simulink model "Autotrans_shift3"  (R2024a)
settings: Solver=VariableStepAuto  StartTime=0.0  StopTime=35.0  RelTol=0.001
model workspace (MATLAB code in the model file):
  | load sldemo_autotrans_data; %load initial conditions and other necessary data
undefined symbols (not defined in the file or in its folder): converter_data, downtab, emap, Hecate_brake1, Hecate_brake2, Hecate_throttle1, Hecate_throttle2, Hecate_trans, Iei, uptab, vehicledata
(part 1 of 2)
settings Model: DataTypeOverride=Off  MinMaxOverflowLogging=ForceOff  SimulationMode=accelerator  LastModifiedBy=fedformi_new
settings SolverCC: ConsecutiveZCsStepRelTol=2.8421709430404e-13
settings DataIOCC: SaveFormat=Array
settings OptimizationCC: BlockReduction=off  BooleanDataType=off  ReuseModelBlockBuffer=off
settings DebuggingCC: SaveWithParameterizedLinksMsg=none  UnderspecifiedInitializationDetection=Classic  MergeDetectMultiDrivingBlocksExec=none  SignalResolutionControl=TryResolveAllWithWarning
settings HardwareCC: TargetUnknown=on
settings ModelReferenceCC: PropagateSignalLabelsOutOfModel=off
settings RTWCC: GPUComputeCapability=3.5

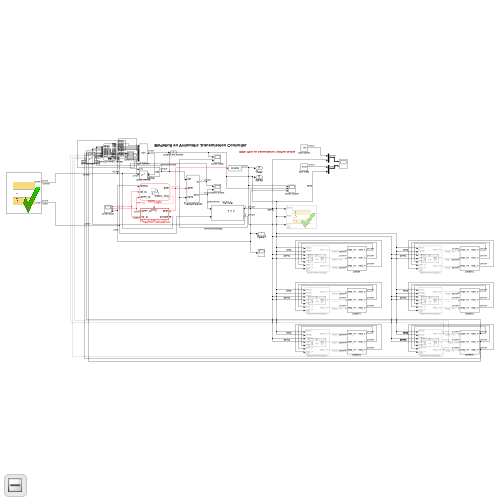
[thumbnail: Simulink's stored preview of the top-level diagram]
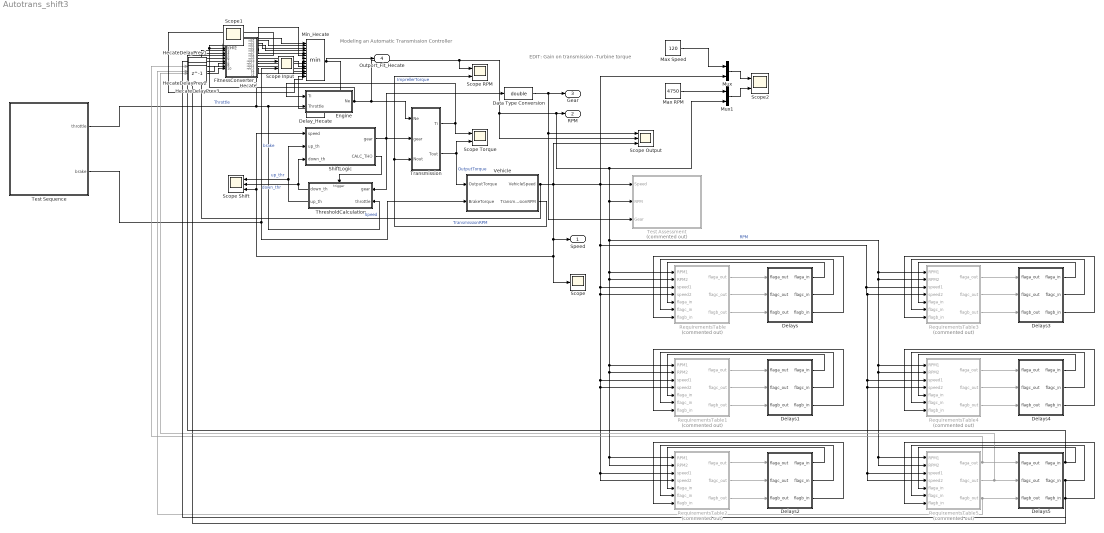
== system Autotrans_shift3 ==
  note: EDIT: Gain on transmission -Turbine torque
  note: Modeling an Automatic Transmission Controller
  Data Type Conversion : DataTypeConversion  OutDataTypeStr=double  SaturateOnIntegerOverflow=off  RndMeth=Floor
  Delay_Hecate : Delay  DelayLength=1  InitialCondition=Inf
  Delays : Subsystem
  Delays1 : Subsystem
  Delays2 : Subsystem
  Delays3 : Subsystem
  Delays4 : Subsystem
  Delays5 : Subsystem
  Engine : Subsystem
  FitnessConverter_Hecate : Stateflow chart  TreatAsAtomicUnit=on
  HecateDelayPrev1 : Delay  DelayLength=1  InitialCondition=0
  HecateDelayPrev2 : Delay  DelayLength=1  InitialCondition=0
  HecateDelayPrev3 : Delay  DelayLength=1  InitialCondition=0
  Max RPM : Constant  Value=4750
  Max Speed : Constant  Value=120
  Min_Hecate : MinMax  Inputs=14
  Mux : Mux  Inputs=2
  Mux1 : Mux  Inputs=2
  RequirementsTable : Requirements Table  Commented=on  TreatAsAtomicUnit=on
  RequirementsTable1 : Requirements Table  Commented=on  TreatAsAtomicUnit=on
  RequirementsTable2 : Requirements Table  Commented=on  TreatAsAtomicUnit=on
  RequirementsTable3 : Requirements Table  Commented=on  TreatAsAtomicUnit=on
  RequirementsTable4 : Requirements Table  Commented=on  TreatAsAtomicUnit=on
  RequirementsTable5 : Requirements Table  Commented=on  TreatAsAtomicUnit=on
  Scope : Scope
  Scope Input : Scope  NumInputPorts=2
  Scope Output : Scope  NumInputPorts=3
  Scope RPM : Scope  NumInputPorts=2
  Scope Shift : Scope  NumInputPorts=3
  Scope Torque : Scope  NumInputPorts=2
  Scope2 : Scope  NumInputPorts=2
  ShiftLogic : Stateflow chart  TreatAsAtomicUnit=on
  Test Assessment : Test Sequence  Commented=on  TreatAsAtomicUnit=on
  Test Sequence : Test Sequence  TreatAsAtomicUnit=on
  ThresholdCalculation : Subsystem  TreatAsAtomicUnit=on
  Transmission : Subsystem
  Vehicle : Subsystem  mask(vehicle model){Rfd=vehicledata(1), rload0=vehicledata(2), rload2=vehicledata(3), Rw=vehicledata(4), Iv=vehicledata(5), N20=vehicledata(6)/vehicledata(4)*vehicledata(1)}
      mask prompts: Rfd "final drive ratio"; rload0 "drag friction at wheels"; rload2 "aerodynamic drag"; Rw "wheel radius"; Iv "vehicle inertia"; N20 "initial transmission output speed"
      mask help: vehicle dynamics: torque input from trans., outputs are input speed (transmission output) and vehicle speed
      mask Display: image(imread([matlabroot,'/toolbox/simulink/simdemos/automotive/html/NSX_3Colors.jpg']))
  Speed : Outport  VectorParamsAs1DForOutWhenUnconnected=off
  RPM : Outport  Port=2  VectorParamsAs1DForOutWhenUnconnected=off
  Gear : Outport  Port=3  VectorParamsAs1DForOutWhenUnconnected=off
  Outport_Fit_Hecate : Outport  Port=4
  Scope1 : Scope
  wires:
  Transmission/1(Ti) -> Engine/1(Ti), Scope Torque/1  "ImprellerTorque"
  Vehicle/2(TransmissionRPM) -> Transmission/3(Nout), Scope RPM/2  "TransmissionRPM"
  ThresholdCalculation/1(down_th) -> Scope Shift/2, ShiftLogic/3(down_th)  "down_thr"
  ThresholdCalculation/2(up_th) -> ShiftLogic/2(up_th), Scope Shift/1  "up_thr"
  ShiftLogic/1(gear) -> Transmission/2(gear), ThresholdCalculation/1(gear), Data Type Conversion/1
  ShiftLogic/2(CALC_TH()) -> ThresholdCalculation/Trigger
  Test Sequence/1(throttle) -> Engine/2(Throttle), ThresholdCalculation/2(throttle), Scope Input/1  "Throttle"
  Transmission/2(Tout) -> Vehicle/1(OutputTorque), Scope Torque/2  "OutputTorque"
  Test Sequence/2(brake) -> Vehicle/2(BrakeTorque), Scope Input/2  "brake"
  Data Type Conversion/1 -> Scope Output/1, Test Assessment/3(Gear), Gear/1
  Mux1/1 -> Scope2/2
  Max RPM/1 -> Mux1/1
  Max Speed/1 -> Mux/1
  Mux/1 -> Scope2/1
  Delays4/1(flaga_in) -> RequirementsTable4/5(flaga_in)
  RequirementsTable1/2(flagc_out) -> Delays1/2(flagc_out)
  RequirementsTable4/2(flagc_out) -> Delays4/2(flagc_out)
  Delays4/2(flagc_in) -> RequirementsTable4/6(flagc_in)
  Delays1/2(flagc_in) -> RequirementsTable1/6(flagc_in)
  RequirementsTable4/1(flaga_out) -> Delays4/1(flaga_out)
  Vehicle/1(VehicleSpeed) -> FitnessConverter_Hecate/3(speed1), FitnessConverter_Hecate/4(speed2), Speed/1, Scope/1, Scope Shift/3, ShiftLogic/1(speed), Mux/2, Test Assessment/1(Speed), RequirementsTable3/3(speed1), RequirementsTable3/4(speed2), RequirementsTable4/3(speed1), RequirementsTable4/4(speed2), RequirementsTable5/3(speed1), RequirementsTable5/4(speed2), RequirementsTable/3(speed1), RequirementsTable/4(speed2), RequirementsTable1/3(speed1), RequirementsTable1/4(speed2), RequirementsTable2/3(speed1), RequirementsTable2/4(speed2), Scope Output/3  "Speed"
  RequirementsTable/3(flagb_out) -> Delays/3(flagb_out)
  RequirementsTable2/3(flagb_out) -> Delays2/3(flagb_out)
  RequirementsTable3/2(flagc_out) -> Delays3/2(flagc_out)
  Delays2/3(flagb_in) -> RequirementsTable2/7(flagb_in)
  RequirementsTable4/3(flagb_out) -> Delays4/3(flagb_out)
  Delays/1(flaga_in) -> RequirementsTable/5(flaga_in)
  RequirementsTable1/3(flagb_out) -> Delays1/3(flagb_out)
  Delays4/3(flagb_in) -> RequirementsTable4/7(flagb_in)
  Delays/2(flagc_in) -> RequirementsTable/6(flagc_in)
  RequirementsTable5/3(flagb_out) -> Delays5/3(flagb_out), HecateDelayPrev2/1
  Delays2/1(flaga_in) -> RequirementsTable2/5(flaga_in)
  Delays1/1(flaga_in) -> RequirementsTable1/5(flaga_in)
  RequirementsTable2/2(flagc_out) -> Delays2/2(flagc_out)
  Delays1/3(flagb_in) -> RequirementsTable1/7(flagb_in)
  RequirementsTable/2(flagc_out) -> Delays/2(flagc_out)
  RequirementsTable5/1(flaga_out) -> Delays5/1(flaga_out), HecateDelayPrev1/1
  Delays/3(flagb_in) -> RequirementsTable/7(flagb_in)
  RequirementsTable1/1(flaga_out) -> Delays1/1(flaga_out)
  RequirementsTable/1(flaga_out) -> Delays/1(flaga_out)
  Delays2/2(flagc_in) -> RequirementsTable2/6(flagc_in)
  Delays3/2(flagc_in) -> RequirementsTable3/6(flagc_in)
  RequirementsTable2/1(flaga_out) -> Delays2/1(flaga_out)
  Engine/1(Ne) -> FitnessConverter_Hecate/1(RPM1), FitnessConverter_Hecate/2(RPM2), Transmission/1(Ne), Scope RPM/1, Mux1/2, RequirementsTable3/1(RPM1), RequirementsTable3/2(RPM2), RequirementsTable4/1(RPM1), RequirementsTable4/2(RPM2), RequirementsTable5/1(RPM1), RequirementsTable5/2(RPM2), RequirementsTable/1(RPM1), RequirementsTable/2(RPM2), RequirementsTable1/1(RPM1), RequirementsTable1/2(RPM2), RequirementsTable2/1(RPM1), RequirementsTable2/2(RPM2), Test Assessment/2(RPM), RPM/1, Scope Output/2  "RPM"
  Delays5/2(flagc_in) -> RequirementsTable5/6(flagc_in), FitnessConverter_Hecate/6(flagc_in)
  Delays3/3(flagb_in) -> RequirementsTable3/7(flagb_in)
  RequirementsTable5/2(flagc_out) -> Delays5/2(flagc_out), HecateDelayPrev3/1
  Delays5/3(flagb_in) -> RequirementsTable5/7(flagb_in), FitnessConverter_Hecate/7(flagb_in)
  Delays5/1(flaga_in) -> RequirementsTable5/5(flaga_in), FitnessConverter_Hecate/5(flaga_in)
  RequirementsTable3/3(flagb_out) -> Delays3/3(flagb_out)
  RequirementsTable3/1(flaga_out) -> Delays3/1(flaga_out)
  Delays3/1(flaga_in) -> RequirementsTable3/5(flaga_in)
  HecateDelayPrev1/1 -> FitnessConverter_Hecate/8(flaga_outPrev)
  HecateDelayPrev2/1 -> FitnessConverter_Hecate/9(flagb_outPrev)
  HecateDelayPrev3/1 -> FitnessConverter_Hecate/10(flagc_outPrev)
  FitnessConverter_Hecate/1(rob1) -> Min_Hecate/1
  FitnessConverter_Hecate/2(rob2) -> Min_Hecate/2
  FitnessConverter_Hecate/3(rob3) -> Min_Hecate/3
  FitnessConverter_Hecate/4(rob4) -> Min_Hecate/4
  FitnessConverter_Hecate/5(rob5) -> Min_Hecate/5
  FitnessConverter_Hecate/6(rob6) -> Min_Hecate/6
  FitnessConverter_Hecate/7(rob7) -> Min_Hecate/7
  FitnessConverter_Hecate/8(rob8) -> Min_Hecate/8
  FitnessConverter_Hecate/9(rob9) -> Min_Hecate/9
  FitnessConverter_Hecate/10(rob10) -> Min_Hecate/10
  FitnessConverter_Hecate/11(rob11) -> Min_Hecate/11
  FitnessConverter_Hecate/12(rob12) -> Min_Hecate/12
  FitnessConverter_Hecate/13(rob13) -> Min_Hecate/13
  Min_Hecate/1 -> Delay_Hecate/1, Outport_Fit_Hecate/1
  Delay_Hecate/1 -> Min_Hecate/14

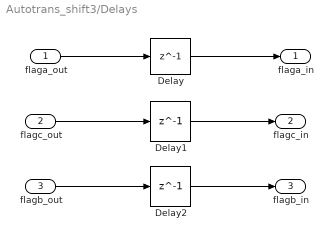
== system Autotrans_shift3/Delays ==
  flaga_out : Inport  OutDataTypeStr=boolean
  flagc_out : Inport  Port=2  OutDataTypeStr=boolean
  flagb_out : Inport  Port=3  OutDataTypeStr=boolean
  Delay : Delay  DelayLength=1  InitialCondition=false  UseCircularBuffer=on
  Delay1 : Delay  DelayLength=1  InitialCondition=false  UseCircularBuffer=on
  Delay2 : Delay  DelayLength=1  InitialCondition=false  UseCircularBuffer=on
  flaga_in : Outport  OutDataTypeStr=boolean
  flagc_in : Outport  Port=2  OutDataTypeStr=boolean
  flagb_in : Outport  Port=3  OutDataTypeStr=boolean
  wires:
  flaga_out/1 -> Delay/1
  Delay/1 -> flaga_in/1
  flagc_out/1 -> Delay1/1
  Delay1/1 -> flagc_in/1
  flagb_out/1 -> Delay2/1
  Delay2/1 -> flagb_in/1

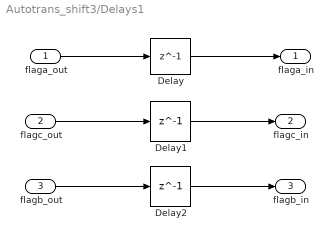
== system Autotrans_shift3/Delays1 ==
  flaga_out : Inport  OutDataTypeStr=boolean
  flagc_out : Inport  Port=2  OutDataTypeStr=boolean
  flagb_out : Inport  Port=3  OutDataTypeStr=boolean
  Delay : Delay  DelayLength=1  InitialCondition=false  UseCircularBuffer=on
  Delay1 : Delay  DelayLength=1  InitialCondition=false  UseCircularBuffer=on
  Delay2 : Delay  DelayLength=1  InitialCondition=false  UseCircularBuffer=on
  flaga_in : Outport  OutDataTypeStr=boolean
  flagc_in : Outport  Port=2  OutDataTypeStr=boolean
  flagb_in : Outport  Port=3  OutDataTypeStr=boolean
  wires:
  flaga_out/1 -> Delay/1
  Delay/1 -> flaga_in/1
  flagc_out/1 -> Delay1/1
  Delay1/1 -> flagc_in/1
  flagb_out/1 -> Delay2/1
  Delay2/1 -> flagb_in/1

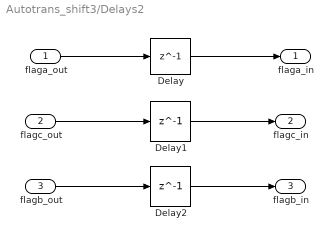
== system Autotrans_shift3/Delays2 ==
  flaga_out : Inport  OutDataTypeStr=boolean
  flagc_out : Inport  Port=2  OutDataTypeStr=boolean
  flagb_out : Inport  Port=3  OutDataTypeStr=boolean
  Delay : Delay  DelayLength=1  InitialCondition=false  UseCircularBuffer=on
  Delay1 : Delay  DelayLength=1  InitialCondition=false  UseCircularBuffer=on
  Delay2 : Delay  DelayLength=1  InitialCondition=false  UseCircularBuffer=on
  flaga_in : Outport  OutDataTypeStr=boolean
  flagc_in : Outport  Port=2  OutDataTypeStr=boolean
  flagb_in : Outport  Port=3  OutDataTypeStr=boolean
  wires:
  flaga_out/1 -> Delay/1
  Delay/1 -> flaga_in/1
  flagc_out/1 -> Delay1/1
  Delay1/1 -> flagc_in/1
  flagb_out/1 -> Delay2/1
  Delay2/1 -> flagb_in/1

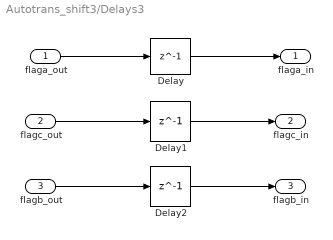
== system Autotrans_shift3/Delays3 ==
  flaga_out : Inport  OutDataTypeStr=boolean
  flagc_out : Inport  Port=2  OutDataTypeStr=boolean
  flagb_out : Inport  Port=3  OutDataTypeStr=boolean
  Delay : Delay  DelayLength=1  InitialCondition=false  UseCircularBuffer=on
  Delay1 : Delay  DelayLength=1  InitialCondition=false  UseCircularBuffer=on
  Delay2 : Delay  DelayLength=1  InitialCondition=false  UseCircularBuffer=on
  flaga_in : Outport  OutDataTypeStr=boolean
  flagc_in : Outport  Port=2  OutDataTypeStr=boolean
  flagb_in : Outport  Port=3  OutDataTypeStr=boolean
  wires:
  flaga_out/1 -> Delay/1
  Delay/1 -> flaga_in/1
  flagc_out/1 -> Delay1/1
  Delay1/1 -> flagc_in/1
  flagb_out/1 -> Delay2/1
  Delay2/1 -> flagb_in/1

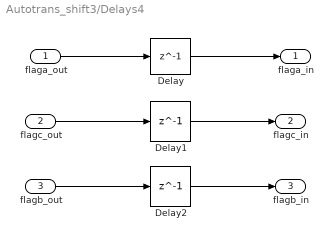
== system Autotrans_shift3/Delays4 ==
  flaga_out : Inport  OutDataTypeStr=boolean
  flagc_out : Inport  Port=2  OutDataTypeStr=boolean
  flagb_out : Inport  Port=3  OutDataTypeStr=boolean
  Delay : Delay  DelayLength=1  InitialCondition=false  UseCircularBuffer=on
  Delay1 : Delay  DelayLength=1  InitialCondition=false  UseCircularBuffer=on
  Delay2 : Delay  DelayLength=1  InitialCondition=false  UseCircularBuffer=on
  flaga_in : Outport  OutDataTypeStr=boolean
  flagc_in : Outport  Port=2  OutDataTypeStr=boolean
  flagb_in : Outport  Port=3  OutDataTypeStr=boolean
  wires:
  flaga_out/1 -> Delay/1
  Delay/1 -> flaga_in/1
  flagc_out/1 -> Delay1/1
  Delay1/1 -> flagc_in/1
  flagb_out/1 -> Delay2/1
  Delay2/1 -> flagb_in/1

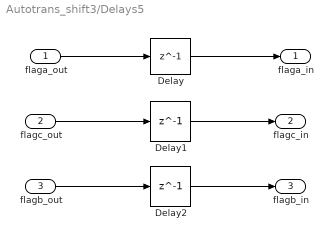
== system Autotrans_shift3/Delays5 ==
  flaga_out : Inport  OutDataTypeStr=boolean
  flagc_out : Inport  Port=2  OutDataTypeStr=boolean
  flagb_out : Inport  Port=3  OutDataTypeStr=boolean
  Delay : Delay  DelayLength=1  InitialCondition=false  UseCircularBuffer=on
  Delay1 : Delay  DelayLength=1  InitialCondition=false  UseCircularBuffer=on
  Delay2 : Delay  DelayLength=1  InitialCondition=false  UseCircularBuffer=on
  flaga_in : Outport  OutDataTypeStr=boolean
  flagc_in : Outport  Port=2  OutDataTypeStr=boolean
  flagb_in : Outport  Port=3  OutDataTypeStr=boolean
  wires:
  flaga_out/1 -> Delay/1
  Delay/1 -> flaga_in/1
  flagc_out/1 -> Delay1/1
  Delay1/1 -> flagc_in/1
  flagb_out/1 -> Delay2/1
  Delay2/1 -> flagb_in/1

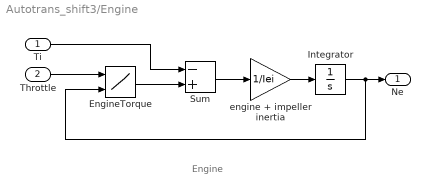
== system Autotrans_shift3/Engine ==
  note: Engine
  Ti : Inport
  Throttle : Inport  Port=2
  EngineTorque : Lookup2D  RowIndex=thvec  ColumnIndex=nevec  Table=emap  SaturateOnIntegerOverflow=off
  Integrator : Integrator  InitialCondition=1000  LimitOutput=on  UpperSaturationLimit=6000  LowerSaturationLimit=600  ZeroCross=off
  Sum : Sum  Inputs=-+  InputSameDT=on  SaturateOnIntegerOverflow=on  OutDataTypeStr=Inherit: Same as first input
  engine + impeller inertia : Gain  Gain=1/Iei  SaturateOnIntegerOverflow=on  OutDataTypeStr=Inherit: Same as input  ParamDataTypeStr=Inherit: Same as input
  Ne : Outport  InitialOutput=0  VectorParamsAs1DForOutWhenUnconnected=off
  wires:
  Ti/1 -> Sum/1
  Throttle/1 -> EngineTorque/1
  Integrator/1 -> EngineTorque/2, Ne/1
  Sum/1 -> engine + impeller inertia/1
  engine + impeller inertia/1 -> Integrator/1
  EngineTorque/1 -> Sum/2

== system Autotrans_shift3/ThresholdCalculation ==
  note: Threshold Calculation
  gear : Inport
  throttle : Inport  Port=2
  run : TriggerPort  TriggerType=function-call  VariantControl=(inherit)  ZeroCross=off
  interp_down : Lookup2D  RowIndex=downth  ColumnIndex=[1:4]  Table=downtab  OutDataTypeStr=double  SaturateOnIntegerOverflow=off  InputSameDT=off
      settings: LockScale=on
  interp_up : Lookup2D  RowIndex=upth  ColumnIndex=[1:4]  Table=uptab  OutDataTypeStr=double  SaturateOnIntegerOverflow=off  InputSameDT=off
      settings: LockScale=on
  down_th : Outport  VectorParamsAs1DForOutWhenUnconnected=off
  up_th : Outport  Port=2  VectorParamsAs1DForOutWhenUnconnected=off
  wires:
  interp_up/1 -> up_th/1
  interp_down/1 -> down_th/1
  throttle/1 -> interp_up/1, interp_down/1
  gear/1 -> interp_up/2, interp_down/2

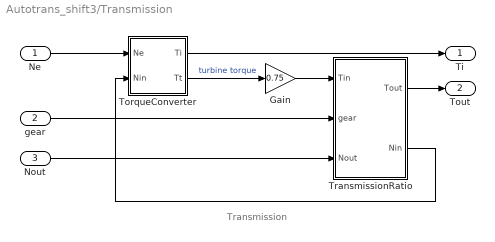
== system Autotrans_shift3/Transmission ==
  note: Transmission
  Ne : Inport
  gear : Inport  Port=2
  Nout : Inport  Port=3
  Gain : Gain  Gain=0.75
  TorqueConverter : Subsystem  mask(torque converter){speedratio=converter_data(:,1), Kfactor=converter_data(:,2), Torkratio=converter_data(:,3)}
      mask prompts: speedratio "speed ratio"; Kfactor "K factor"; Torkratio "torque ratio"
      mask help: torque converter
      mask Help: Torque converter input and output torques are computed as a function of the input and output speeds
      mask Display: plot([cos([90:10:450]*pi/180),.63*cos([90:10:450]*pi/180),.63*cos([90:10:240]*pi/180),cos([240:10:300]*pi/180),.63*cos([300]*pi/180)],[sin([90:10:450]*pi/180),.63*sin([90:10:450]*pi/180)+.1,.63*sin([90:10:240]*pi/180)+.1,sin([240:10:300]*pi/180),.63*sin([300]*pi/180)+.1])
  TransmissionRatio : Subsystem
  Ti : Outport  InitialOutput=0  VectorParamsAs1DForOutWhenUnconnected=off
  Tout : Outport  Port=2  InitialOutput=0  VectorParamsAs1DForOutWhenUnconnected=off
  wires:
  TransmissionRatio/1(Tout) -> Tout/1
  TorqueConverter/1(Ti) -> Ti/1
  Nout/1 -> TransmissionRatio/3(Nout)
  gear/1 -> TransmissionRatio/2(gear)
  Ne/1 -> TorqueConverter/1(Ne)
  TransmissionRatio/2(Nin) -> TorqueConverter/2(Nin)
  TorqueConverter/2(Tt) -> Gain/1  "turbine torque"
  Gain/1 -> TransmissionRatio/1(Tin)

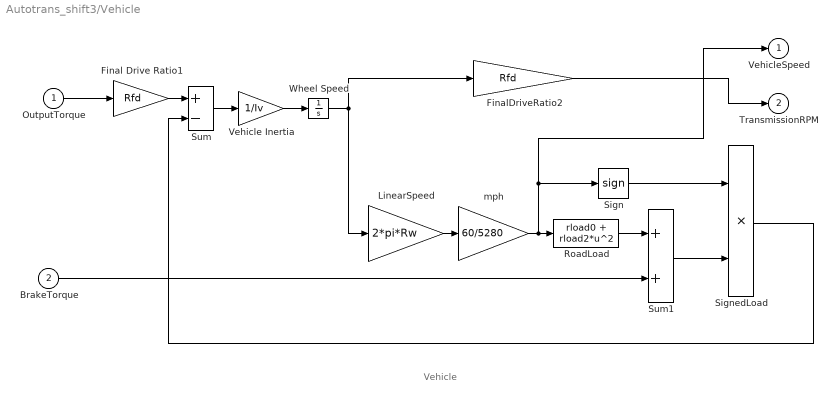
== system Autotrans_shift3/Vehicle ==
  note: Vehicle
  OutputTorque : Inport
  BrakeTorque : Inport  Port=2
  Final Drive Ratio1 : Gain  Gain=Rfd  SaturateOnIntegerOverflow=on  OutDataTypeStr=Inherit: Same as input  ParamDataTypeStr=Inherit: Same as input
  FinalDriveRatio2 : Gain  Gain=Rfd  SaturateOnIntegerOverflow=on  OutDataTypeStr=Inherit: Same as input  ParamDataTypeStr=Inherit: Same as input
  LinearSpeed : Gain  Gain=2*pi*Rw  SaturateOnIntegerOverflow=on  OutDataTypeStr=Inherit: Same as input  ParamDataTypeStr=Inherit: Same as input
  RoadLoad : Fcn  Expr=rload0 + rload2*u^2
  Sign : Signum
  SignedLoad : Product  InputSameDT=on  SaturateOnIntegerOverflow=on  OutDataTypeStr=Inherit: Same as first input
  Sum : Sum  Inputs=+-  InputSameDT=on  SaturateOnIntegerOverflow=on  OutDataTypeStr=Inherit: Same as first input
  Sum1 : Sum  InputSameDT=on  SaturateOnIntegerOverflow=on  OutDataTypeStr=Inherit: Same as first input
  Vehicle Inertia : Gain  Gain=1/Iv  SaturateOnIntegerOverflow=on  OutDataTypeStr=Inherit: Same as input  ParamDataTypeStr=Inherit: Same as input
  Wheel Speed : Integrator  InitialCondition=N20/Rfd  ZeroCross=off
  mph : Gain  Gain=60/5280  SaturateOnIntegerOverflow=on  OutDataTypeStr=Inherit: Same as input  ParamDataTypeStr=Inherit: Same as input
  VehicleSpeed : Outport  InitialOutput=0  VectorParamsAs1DForOutWhenUnconnected=off
  TransmissionRPM : Outport  Port=2  InitialOutput=0  VectorParamsAs1DForOutWhenUnconnected=off
  wires:
  FinalDriveRatio2/1 -> TransmissionRPM/1
  BrakeTorque/1 -> Sum1/2
  Sum1/1 -> SignedLoad/2
  RoadLoad/1 -> Sum1/1
  Sign/1 -> SignedLoad/1
  SignedLoad/1 -> Sum/2
  OutputTorque/1 -> Final Drive Ratio1/1
  Vehicle Inertia/1 -> Wheel Speed/1
  Sum/1 -> Vehicle Inertia/1
  mph/1 -> VehicleSpeed/1, Sign/1, RoadLoad/1
  LinearSpeed/1 -> mph/1
  Wheel Speed/1 -> LinearSpeed/1, FinalDriveRatio2/1
  Final Drive Ratio1/1 -> Sum/1

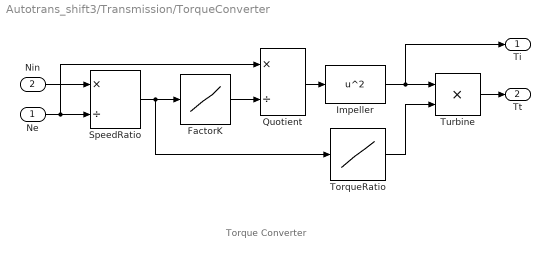
== system Autotrans_shift3/Transmission/TorqueConverter ==
  note: Torque Converter
  Ne : Inport
  Nin : Inport  Port=2
  FactorK : Lookup  InputValues=speedratio  Table=Kfactor
  Impeller : Fcn  Expr=u^2
  Quotient : Product  Inputs=*/  InputSameDT=on  SaturateOnIntegerOverflow=on  OutDataTypeStr=Inherit: Same as first input
  SpeedRatio : Product  Inputs=*/  InputSameDT=on  SaturateOnIntegerOverflow=on  OutDataTypeStr=Inherit: Same as first input
  TorqueRatio : Lookup  InputValues=speedratio  Table=Torkratio
  Turbine : Product  InputSameDT=on  SaturateOnIntegerOverflow=on  OutDataTypeStr=Inherit: Same as first input
  Ti : Outport  InitialOutput=0  VectorParamsAs1DForOutWhenUnconnected=off
  Tt : Outport  Port=2  InitialOutput=0  VectorParamsAs1DForOutWhenUnconnected=off
  wires:
  TorqueRatio/1 -> Turbine/2
  Quotient/1 -> Impeller/1
  FactorK/1 -> Quotient/2
  SpeedRatio/1 -> TorqueRatio/1, FactorK/1
  Impeller/1 -> Turbine/1, Ti/1
  Turbine/1 -> Tt/1
  Ne/1 -> SpeedRatio/2, Quotient/1
  Nin/1 -> SpeedRatio/1

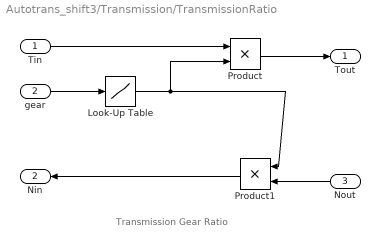
== system Autotrans_shift3/Transmission/TransmissionRatio ==
  note: Transmission Gear Ratio
  Tin : Inport
  gear : Inport  Port=2
  Nout : Inport  Port=3
  Look-Up Table : Lookup  InputValues=[1 2 3 4]  Table=[2.393 1.450 1.000 0.677]  OutDataTypeStr=double  LockScale=on
  Product : Product  InputSameDT=on  SaturateOnIntegerOverflow=on  OutDataTypeStr=Inherit: Same as first input
  Product1 : Product  InputSameDT=on  SaturateOnIntegerOverflow=on  OutDataTypeStr=Inherit: Same as first input
  Tout : Outport  InitialOutput=0  VectorParamsAs1DForOutWhenUnconnected=off
  Nin : Outport  Port=2  InitialOutput=0  VectorParamsAs1DForOutWhenUnconnected=off
  wires:
  Look-Up Table/1 -> Product1/1, Product/2
  Nout/1 -> Product1/2
  Product1/1 -> Nin/1
  Product/1 -> Tout/1
  Tin/1 -> Product/1
  gear/1 -> Look-Up Table/1

== stateflow chart Autotrans_shift3/ShiftLogic ==
  settings: updateMethod=DISCRETE  sampleTime=0.04
  state gear_state [parallel]
    settings: executionOrder=1
    state fourth
      entry:
      gear = 4;
    state third
      entry:
      gear = 3;
    state second
      entry:
      gear = 2;
    state first
      entry:
      gear = 1;
    (default) -> first
    second -> third [order 1] : UP
    first -> second : UP
    third -> fourth [order 1] : UP
    second -> first [order 2] : DOWN
    fourth -> third : DOWN
    third -> second [order 2] : DOWN
  state selection_state [parallel]
    during: CALC_TH;
    settings: executionOrder=2
    state steady_state
    state upshifting
    state downshifting
    (default) -> steady_state
    steady_state -> upshifting [order 1] : [speed > up_th]
    steady_state -> downshifting [order 2] : [speed < down_th]
    downshifting -> steady_state [order 1] : after(TWAIT,tick)
        | [speed <= down_th]
        | {gear_state.DOWN;}
    downshifting -> steady_state [order 2] : [speed > down_th]
    upshifting -> steady_state [order 1] : after(TWAIT,tick)
        | [speed >= up_th]
        | {gear_state.UP;}
    upshifting -> steady_state [order 2] : [speed < up_th]
  data: speed input double; gear output fixdt(0,8,5) [1..4]; TWAIT parameter fixdt(0,8,6); up_th input double; down_th input double
  events: DOWN local EITHER_EDGE_EVENT; UP local EITHER_EDGE_EVENT; CALC_TH output FUNCTION_CALL_EVENT

== stateflow chart Autotrans_shift3/Test Assessment ==
  state AT1
    state step_1
      state step_1_1
        verify(Speed < 120);
        settings: description=|
            | the value of the speed between [0,20]s
            | shall be lower than 120mph
      state step_1_2
      AT1.step_1 -> (junction 405)
      (default) -> (junction 405)
      (junction 405) -> (junction 406) [order 1] : [((t>=0) && (t<=20))
          | ]
      (junction 406) -> AT1.step_1.step_1_1 [order 1] : [~in(AT1.step_1.step_1_1)]
      (junction 406) -> (junction 409) [order 2]
      (junction 725) -> (junction 726)
      (junction 726) -> AT1.step_1.step_1_2 [order 1] : [~in(AT1.step_1.step_1_2)]
      (junction 726) -> (junction 729) [order 2]
      (junction 405) -> (junction 725) [order 2]
    (default) -> AT1.step_1
  state AT2
    state step_1
      state step_1_1
        verify(RPM<4750, 'Message')
      state step_1_2
      (default) -> (junction 433)
      AT2.step_1 -> (junction 433)
      (junction 433) -> (junction 434) [order 1] : [(t>=0 && t<=10)
          | ]
      (junction 434) -> AT2.step_1.step_1_1 [order 1] : [~in(AT2.step_1.step_1_1)]
      (junction 433) -> (junction 733) [order 2]
      (junction 434) -> (junction 437) [order 2]
      (junction 733) -> (junction 734)
      (junction 734) -> AT2.step_1.step_1_2 [order 1] : [~in(AT2.step_1.step_1_2)]
      (junction 734) -> (junction 737) [order 2]
    (default) -> AT2.step_1
  state AT51
    state step_1
    state AT51
      settings: description=Trigger upon changing to gear 1
    state AT51_1
      verify(Gear==1)
    (default) -> AT51.step_1
    AT51.AT51 -> AT51_1 : [
        | (hasChangedTo(Gear,1) && t>=0 && t<=30)
        | ]
    AT51_1 -> AT51.AT51 : [
        | et > 2.5
        | ]
    AT51.step_1 -> AT51.AT51 : [
        | Gear~=1
        | ]
  state AT52
    state AT52
      settings: description=Trigger upon changing to gear 2
    state AT52_1
      verify(Gear==2)
    (default) -> AT52.AT52
    AT52.AT52 -> AT52_1 : [
        | (hasChangedTo(Gear,2) && t>=0 && t<=30)
        | ]
    AT52_1 -> AT52.AT52 : [
        | et > 2.5
        | ]
  state AT53
    state AT53
      settings: description=Trigger upon changing to gear 3
    state AT53_1
      verify(Gear==3)
    (default) -> AT53.AT53
    AT53.AT53 -> AT53_1 : [
        | (hasChangedTo(Gear,3) && t>=0 && t<=30)
        | ]
    AT53_1 -> AT53.AT53 : [
        | et > 2.5
        | ]
  state AT54
    state AT54
      settings: description=Trigger upon changing to gear 4
    state AT54_1
      verify(Gear==4)
    (default) -> AT54.AT54
    AT54.AT54 -> AT54_1 : [
        | (hasChangedTo(Gear,4) && t>=0 && t<=30)
        | ]
    AT54_1 -> AT54.AT54 : [
        | et > 2.5
        | ]
  state AT6a
    state step_1
    state step_2_Inconclusive
    state step_3
    state step_4
    state step_5
      verify(true)
      settings: description=robustness calculation
    state step_6
      verify(false)
    (default) -> AT6a.step_1
    AT6a.step_1 -> (junction 589) [order 2] : [
        | ~(Speed<35)
        | ]
    (junction 589) -> (junction 587)
    AT6a.step_1 -> (junction 593) [order 3] : [
        | t>=4
        | ]
    (junction 593) -> (junction 591)
    AT6a.step_1 -> AT6a.step_2_Inconclusive [order 1] : [
        | ~(RPM<3000)
        | ]
    (junction 608) -> AT6a.step_2_Inconclusive
    (junction 610) -> (junction 608)
    AT6a.step_3 -> AT6a.step_2_Inconclusive [order 1] : [
        | ~(RPM<3000)
        | ]
    (junction 587) -> AT6a.step_3
    AT6a.step_3 -> (junction 758) [order 2] : [
        | t>=30
        | ]
    (junction 758) -> (junction 601)
    AT6a.step_4 -> (junction 610) [order 1] : [
        | ~(RPM<3000)
        | ]
    (junction 591) -> AT6a.step_4
    AT6a.step_4 -> (junction 619) [order 2] : [
        | t>=30
        | ]
    (junction 619) -> (junction 612)
    (junction 601) -> AT6a.step_5
    (junction 612) -> AT6a.step_6
  state AT6b
    state step_1
    state step_2_Inconclusive
    state step_3
    state step_4
    state step_5
      verify(true)
    state step_6
      verify(false)
    AT6b.step_4 -> (junction 658) [order 2] : [
        | t>=30
        | ]
    (default) -> AT6b.step_1
    AT6b.step_1 -> (junction 634) [order 2] : [
        | ~(Speed<50)
        | ]
    (junction 634) -> (junction 632)
    AT6b.step_1 -> (junction 641) [order 3] : [
        | t>=8
        | ]
    (junction 641) -> (junction 639)
    AT6b.step_1 -> AT6b.step_2_Inconclusive [order 1] : [
        | ~(RPM<3000)
        | ]
    (junction 644) -> AT6b.step_2_Inconclusive
    (junction 646) -> (junction 644)
    AT6b.step_3 -> AT6b.step_2_Inconclusive [order 1] : [
        | ~(RPM<3000)
        | ]
    (junction 632) -> AT6b.step_3
    AT6b.step_3 -> (junction 652) [order 2] : [
        | t>=30
        | ]
    (junction 652) -> (junction 650)
    AT6b.step_4 -> (junction 646) [order 1] : [
        | ~(RPM<3000)
        | ]
    (junction 639) -> AT6b.step_4
    (junction 650) -> AT6b.step_5
    (junction 656) -> AT6b.step_6
    (junction 658) -> (junction 656)
  state AT6c
    state step_1
    state step_2_Inconclusive
    state step_3
    state step_4
    state step_5
      verify(true)
    state step_6
      verify(false)
    AT6c.step_4 -> (junction 698) [order 2] : [
        | t>=30
        | ]
    (default) -> AT6c.step_1
    AT6c.step_1 -> (junction 674) [order 2] : [
        | ~(Speed<65)
        | ]
    (junction 674) -> (junction 672)
    AT6c.step_1 -> (junction 681) [order 3] : [
        | t>=20
        | ]
    (junction 681) -> (junction 679)
    AT6c.step_1 -> AT6c.step_2_Inconclusive [order 1] : [
        | ~(RPM<3000)
        | ]
    (junction 684) -> AT6c.step_2_Inconclusive
    (junction 686) -> (junction 684)
    AT6c.step_3 -> AT6c.step_2_Inconclusive [order 1] : [
        | ~(RPM<3000)
        | ]
    (junction 672) -> AT6c.step_3
    AT6c.step_3 -> (junction 692) [order 2] : [
        | t>=30
        | ]
    (junction 692) -> (junction 690)
    AT6c.step_4 -> (junction 686) [order 1] : [
        | ~(RPM<3000)
        | ]
    (junction 679) -> AT6c.step_4
    (junction 690) -> AT6c.step_5
    (junction 696) -> AT6c.step_6
    (junction 698) -> (junction 696)
  (default) -> AT1 [order 1] : [Active_Scenario_Index == 1]
  (default) -> AT2 [order 2] : [Active_Scenario_Index == 2]
  (default) -> AT51 [order 3] : [Active_Scenario_Index == 3]
  (default) -> AT52 [order 4] : [Active_Scenario_Index == 4]
  (default) -> AT53 [order 5] : [Active_Scenario_Index == 5]
  (default) -> AT54 [order 6] : [Active_Scenario_Index == 6]
  (default) -> AT6a [order 7] : [Active_Scenario_Index == 7]
  (default) -> AT6b [order 8] : [Active_Scenario_Index == 8]
  (default) -> AT6c [order 9] : {assert(Active_Scenario_Index == 9,'The value of Scenario Parameter ''Active_Scenario_Index'' is not valid. Use the index of the scenario to specify it.')}
  data: Speed input; RPM input; Gear input; Active_Scenario_Index parameter =1

== stateflow chart Autotrans_shift3/RequirementsTable1 ==
  (default) -> (junction 1073744871)
  (junction 1073744871) -> (junction 1073744872) : {
      | % SF_REQ_REV_07
      | }
  (junction 1073744872) -> (junction 1073744874) : {
      | % ExcEvals:
      | % PriEvals:
      | }
  (junction 1073744874) -> (junction 1073744876) : {
      | % HEADER_ASSIGNMENTS
      |
      | }
  (junction 1073744876) -> (junction 1073744878) : {
      | % START_A_4
      | }
  (junction 1073744878) -> (junction 1073744880) : {
      | }
  (junction 1073744880) -> (junction 1073744882)
  (junction 1073744882) -> (junction 1073744884) : {
      | }
  (junction 1073744884) -> (junction 1073744886) : {
      | % END_A_4
      | }
  (junction 1073744886) -> (junction 1073744888) : {
      | % START_R_7
      | }
  (junction 1073744888) -> (junction 1073744890) : {
      | }
  (junction 1073744890) -> (junction 1073744892)
  (junction 1073744892) -> (junction 1073744894) [order 1] : [(((t) >= (0) && (t) <= (20)))]
  (junction 1073744892) -> (junction 1073744900) [order 2]
  (junction 1073744894) -> (junction 1073744896) : {
      | reqtable_postcondition(((speed2)/115 < 1), 'R:1');
      |
      |
      |
      |
      | }
  (junction 1073744896) -> (junction 1073744898) : {
      | }
  (junction 1073744898) -> (junction 1073744900)
  (junction 1073744900) -> (junction 1073744902)
  (junction 1073744902) -> (junction 1073744904) : {
      | % END_R_7
      | }
  (junction 1073744904) -> (junction 1073744906) : {
      | % START_R_19
      | }
  (junction 1073744906) -> (junction 1073744908) : {
      | }
  (junction 1073744908) -> (junction 1073744910)
  (junction 1073744910) -> (junction 1073744912) [order 1] : [(((t) >= (0) && (t) <= (10)))]
  (junction 1073744910) -> (junction 1073744918) [order 2]
  (junction 1073744912) -> (junction 1073744914) : {
      | reqtable_postcondition(((RPM2)/4750 < 1), 'R:2');
      |
      |
      |
      |
      | }
  (junction 1073744914) -> (junction 1073744916) : {
      | }
  (junction 1073744916) -> (junction 1073744918)
  (junction 1073744918) -> (junction 1073744920)
  (junction 1073744920) -> (junction 1073744922) : {
      | % END_R_19
      | }
  (junction 1073744922) -> (junction 1073744924) : {
      | % START_R_34
      | }
  (junction 1073744924) -> (junction 1073744926) : {
      | }
  (junction 1073744926) -> (junction 1073744928)
  (junction 1073744928) -> (junction 1073744930) [order 1] : [((t) == 0)]
  (junction 1073744928) -> (junction 1073744936) [order 2]
  (junction 1073744930) -> (junction 1073744932) : {
      | flaga_out = true;
      | flagb_out = true;
      | flagc_out = true;
      |
      | }
  (junction 1073744932) -> (junction 1073744934) : {
      | }
  (junction 1073744934) -> (junction 1073744936)
  (junction 1073744936) -> (junction 1073744938)
  (junction 1073744938) -> (junction 1073744940) : {
      | % END_R_34
      | }
  (junction 1073744940) -> (junction 1073744942) : {
      | % START_R_22
      | }
  (junction 1073744942) -> (junction 1073744944) : {
      | }
  (junction 1073744944) -> (junction 1073744946)
  (junction 1073744946) -> (junction 1073744948) [order 1] : [(((t) <= (4))) && (speed1 >= 32)]
  (junction 1073744946) -> (junction 1073744954) [order 2]
  (junction 1073744948) -> (junction 1073744950) : {
      | flaga_out = false
      |
      |
      |
      | }
  (junction 1073744950) -> (junction 1073744952) : {
      | }
  (junction 1073744952) -> (junction 1073744954)
  (junction 1073744954) -> (junction 1073744956)
  (junction 1073744956) -> (junction 1073744958) : {
      | % END_R_22
      | }
  (junction 1073744958) -> (junction 1073744960) : {
      | % START_R_67
      | }
  (junction 1073744960) -> (junction 1073744962) : {
      | }
  (junction 1073744962) -> (junction 1073744964)
  (junction 1073744964) -> (junction 1073744966) [order 1] : [((t) > 4 || ((t) > 0 && speed1 < 32))]
  (junction 1073744964) -> (junction 1073744972) [order 2]
  (junction 1073744966) -> (junction 1073744968) : {
      | flaga_out = prev(flaga_out);
      |
      |
      |
      | }
  (junction 1073744968) -> (junction 1073744970) : {
      | }
  (junction 1073744970) -> (junction 1073744972)
  (junction 1073744972) -> (junction 1073744974)
  (junction 1073744974) -> (junction 1073744976) : {
      | % END_R_67
      | }
  (junction 1073744976) -> (junction 1073744978) : {
      | % START_R_52
      | }
  (junction 1073744978) -> (junction 1073744980) : {
      | }
  (junction 1073744980) -> (junction 1073744982)
  (junction 1073744982) -> (junction 1073744984) [order 1] : [duration((((t) <= (30))) && (RPM1 < 2900)) >= 30]
  (junction 1073744982) -> (junction 1073744990) [order 2]
  (junction 1073744984) -> (junction 1073744986) : {
      | reqtable_postcondition((((flaga_in) == (true))), 'R:6');
      |
      |
      |
      |
      | }
  (junction 1073744986) -> (junction 1073744988) : {
      | }
  (junction 1073744988) -> (junction 1073744990)
  (junction 1073744990) -> (junction 1073744992)
  (junction 1073744992) -> (junction 1073744994) : {
      | % END_R_52
      | }
  (junction 1073744994) -> (junction 1073744996) : {
      | % START_R_16
      | }
  (junction 1073744996) -> (junction 1073744998) : {
      | }
  (junction 1073744998) -> (junction 1073745000)
  (junction 1073745000) -> (junction 1073745002) [order 1] : [(((t) <= (8))) && (speed1 >= 50)]
  (junction 1073745000) -> (junction 1073745008) [order 2]
  (junction 1073745002) -> (junction 1073745004) : {
      |
      | flagb_out = false;
      |
      |
      | }
  (junction 1073745004) -> (junction 1073745006) : {
      | }
  (junction 1073745006) -> (junction 1073745008)
  (junction 1073745008) -> (junction 1073745010)
  (junction 1073745010) -> (junction 1073745012) : {
      | % END_R_16
      | }
  (junction 1073745012) -> (junction 1073745014) : {
      | % START_R_70
      | }
  (junction 1073745014) -> (junction 1073745016) : {
      | }
  (junction 1073745016) -> (junction 1073745018)
  (junction 1073745018) -> (junction 1073745020) [order 1] : [((t) > 8 || ((t) > 0 && speed1 < 50))]
  (junction 1073745018) -> (junction 1073745026) [order 2]
  (junction 1073745020) -> (junction 1073745022) : {
      |
      | flagb_out = prev(flagb_out);
      |
      |
      | }
  (junction 1073745022) -> (junction 1073745024) : {
      | }
  (junction 1073745024) -> (junction 1073745026)
  (junction 1073745026) -> (junction 1073745028)
  (junction 1073745028) -> (junction 1073745030) : {
      | % END_R_70
      | }
  (junction 1073745030) -> (junction 1073745032) : {
      | % START_R_55
      | }
  (junction 1073745032) -> (junction 1073745034) : {
      | }
  (junction 1073745034) -> (junction 1073745036)
  (junction 1073745036) -> (junction 1073745038) [order 1] : [duration((((t) <= (30))) && (RPM1 < 3000)) >= 30]
  (junction 1073745036) -> (junction 1073745044) [order 2]
  (junction 1073745038) -> (junction 1073745040) : {
      | reqtable_postcondition((((flagb_in) == (true))), 'R:9');
      |
      |
      |
      |
      | }
  (junction 1073745040) -> (junction 1073745042) : {
      | }
  (junction 1073745042) -> (junction 1073745044)
  (junction 1073745044) -> (junction 1073745046)
  (junction 1073745046) -> (junction 1073745048) : {
      | % END_R_55
      | }
  (junction 1073745048) -> (junction 1073745050) : {
      | % START_R_28
      | }
  (junction 1073745050) -> (junction 1073745052) : {
      | }
  (junction 1073745052) -> (junction 1073745054)
  (junction 1073745054) -> (junction 1073745056) [order 1] : [(((t) <= (20))) && (speed1 >= 65)]
  (junction 1073745054) -> (junction 1073745062) [order 2]
  (junction 1073745056) -> (junction 1073745058) : {
      |
      |
      | flagc_out = false;
      |
      | }
  (junction 1073745058) -> (junction 1073745060) : {
      | }
  (junction 1073745060) -> (junction 1073745062)
  (junction 1073745062) -> (junction 1073745064)
  (junction 1073745064) -> (junction 1073745066) : {
      | % END_R_28
      | }
  (junction 1073745066) -> (junction 1073745068) : {
      | % START_R_73
      | }
  (junction 1073745068) -> (junction 1073745070) : {
      | }
  (junction 1073745070) -> (junction 1073745072)
  (junction 1073745072) -> (junction 1073745074) [order 1] : [((t) > 20 || ((t) > 0 && speed1 < 65))]
  (junction 1073745072) -> (junction 1073745080) [order 2]
  (junction 1073745074) -> (junction 1073745076) : {
      |
      |
      | flagc_out = prev(flagc_out);
      |
      | }
  (junction 1073745076) -> (junction 1073745078) : {
      | }
  (junction 1073745078) -> (junction 1073745080)
  (junction 1073745080) -> (junction 1073745082)
  (junction 1073745082) -> (junction 1073745084) : {
      | % END_R_73
      | }
  (junction 1073745084) -> (junction 1073745086) : {
      | % START_R_58
      | }
  (junction 1073745086) -> (junction 1073745088) : {
      | }
  (junction 1073745088) -> (junction 1073745090)
  (junction 1073745090) -> (junction 1073745092) [order 1] : [duration((((t) <= (30))) && (RPM1 < 3000)) >= 30]
  (junction 1073745090) -> (junction 1073745098) [order 2]
  (junction 1073745092) -> (junction 1073745094) : {
      | reqtable_postcondition((((flagc_in) == (true))), 'R:12');
      |
      |
      |
      |
      | }
  (junction 1073745094) -> (junction 1073745096) : {
      | }
  (junction 1073745096) -> (junction 1073745098)
  (junction 1073745098) -> (junction 1073745100)
  (junction 1073745100) -> (junction 1073745102) : {
      | % END_R_58
      | }
  (junction 1073745102) -> (junction 1073745104) : {
      | % START_R_61
      | }
  (junction 1073745104) -> (junction 1073745106) : {
      | }
  (junction 1073745106) -> (junction 1073745108)
  (junction 1073745108) -> (junction 1073745110) [order 1] : [(((t) >= (0) && (t) <= (50)))]
  (junction 1073745108) -> (junction 1073745116) [order 2]
  (junction 1073745110) -> (junction 1073745112) : {
      | reqtable_postcondition((((speed2) >= (0))) && (((RPM2) >= (0))) && ((flaga_in) == true || (flaga_in) == false) && ((flagb_in) == true || (flagb_in) == false) && ((flagc_in) == true || (flagc_in) == false), 'R:13');
      |
      |
      |
      |
      | }
  (junction 1073745112) -> (junction 1073745114) : {
      | }
  (junction 1073745114) -> (junction 1073745116)
  (junction 1073745116) -> (junction 1073745118)
  (junction 1073745118) -> (junction 1073745120) : {
      | % END_R_61
      | }
  data: RPM1 input; RPM2 input; speed1 input; speed2 input; flaga_out output boolean =true; flagc_out output boolean =true; flagb_out output boolean =true; flaga_in input boolean; flagc_in input boolean; flagb_in input boolean

== stateflow chart Autotrans_shift3/Test Sequence ==
  state step_1
    throttle = Hecate_throttle1;
    brake = Hecate_brake1;
  state step_2
    throttle = Hecate_throttle2;
    brake = Hecate_brake2;
  (default) -> step_1
  step_1 -> step_2 : [
      | et > Hecate_trans
      | ]
  data: throttle output; brake output; Hecate_brake2 parameter; Hecate_throttle1 parameter; Hecate_brake1 parameter; Hecate_throttle2 parameter; Hecate_trans parameter

== stateflow chart Autotrans_shift3/FitnessConverter_Hecate ==
  state Requirement_1 [parallel]
    settings: executionOrder=1
    state Default
      rob1 = Inf;
    state Verify
      rob1 = 1-((speed2/125));
    (default) -> (junction 28)
    (junction 28) -> Requirement_1.Verify [order 2]
    (junction 28) -> Requirement_1.Default [order 1] : [~((t>= 0 && t<= 25))]
    Requirement_1.Default -> Requirement_1.Verify : [(t>= 0 && t<= 25)]
    Requirement_1.Verify -> Requirement_1.Default : [~((t>= 0 && t<= 25))]
  state Requirement_2 [parallel]
    settings: executionOrder=2
    state Default
      rob2 = Inf;
    state Verify
      rob2 = 1-((RPM2/4750));
    (default) -> (junction 37)
    (junction 37) -> Requirement_2.Verify [order 2]
    (junction 37) -> Requirement_2.Default [order 1] : [~((t>= 0 && t<= 8))]
    Requirement_2.Default -> Requirement_2.Verify : [(t>= 0 && t<= 8)]
    Requirement_2.Verify -> Requirement_2.Default : [~((t>= 0 && t<= 8))]
  state Requirement_3 [parallel]
    settings: executionOrder=3
    state Default
      rob3 = Inf;
    state Verify
      rob3 = TOKEN_TRUE;
      flaga_out=true;
      flagb_out=true;
      flagc_out=true;
    (default) -> (junction 46)
    (junction 46) -> Requirement_3.Verify [order 2]
    (junction 46) -> Requirement_3.Default [order 1] : [~((t==0))]
    Requirement_3.Default -> Requirement_3.Verify : [(t==0)]
    Requirement_3.Verify -> Requirement_3.Default : [~((t==0))]
  state Requirement_4 [parallel]
    settings: executionOrder=4
    state Default
      rob4 = Inf;
    state Verify
      rob4 = TOKEN_TRUE;
      flaga_out=false;
    (default) -> (junction 56)
    (junction 56) -> Requirement_4.Verify [order 2]
    (junction 56) -> Requirement_4.Default [order 1] : [~((t<=5) && (speed1>=35))]
    Requirement_4.Default -> Requirement_4.Verify : [(t<=5) && (speed1>=35)]
    Requirement_4.Verify -> Requirement_4.Default : [~((t<=5) && (speed1>=35))]
  state Requirement_5 [parallel]
    settings: executionOrder=5
    state Default
      rob5 = Inf;
    state Verify
      rob5 = TOKEN_TRUE;
      flaga_out=flaga_outPrev;
    (default) -> (junction 65)
    (junction 65) -> Requirement_5.Verify [order 2]
    (junction 65) -> Requirement_5.Default [order 1] : [~((t>5||(t>0&&speed1<35)))]
    Requirement_5.Default -> Requirement_5.Verify : [(t>5||(t>0&&speed1<35))]
    Requirement_5.Verify -> Requirement_5.Default : [~((t>5||(t>0&&speed1<35)))]
  state Requirement_6 [parallel]
    settings: executionOrder=6
    state Default
      rob6 = Inf;
    state Wait
      rob6 = Inf;
    state Verify
      rob6 = (flaga_in == true)-abs(flaga_in -( true));
    (default) -> (junction 74)
    (junction 74) -> Requirement_6.Wait [order 2]
    (junction 74) -> Requirement_6.Default [order 1] : [~((t<=30) && (RPM1<3000))]
    Requirement_6.Default -> Requirement_6.Wait : [(t<=30) && (RPM1<3000)]
    Requirement_6.Wait -> Requirement_6.Default [order 1] : [~((t<=30) && (RPM1<3000))]
    Requirement_6.Verify -> Requirement_6.Default : [~((t<=30) && (RPM1<3000))]
    Requirement_6.Wait -> Requirement_6.Verify [order 2] : [et >= 30]
  state Requirement_7 [parallel]
    settings: executionOrder=7
    state Default
      rob7 = Inf;
    state Verify
      rob7 = TOKEN_TRUE;
      flagb_out=false;
    (default) -> (junction 86)
    (junction 86) -> Requirement_7.Verify [order 2]
    (junction 86) -> Requirement_7.Default [order 1] : [~((t<=10) && (speed1>=50))]
    Requirement_7.Default -> Requirement_7.Verify : [(t<=10) && (speed1>=50)]
    Requirement_7.Verify -> Requirement_7.Default : [~((t<=10) && (speed1>=50))]
  state Requirement_8 [parallel]
    settings: executionOrder=8
    state Default
      rob8 = Inf;
    state Verify
      rob8 = TOKEN_TRUE;
      flagb_out=flagb_outPrev;
    (default) -> (junction 95)
    (junction 95) -> Requirement_8.Verify [order 2]
    (junction 95) -> Requirement_8.Default [order 1] : [~((t>10||(t>0&&speed1<50)))]
    Requirement_8.Default -> Requirement_8.Verify : [(t>10||(t>0&&speed1<50))]
    Requirement_8.Verify -> Requirement_8.Default : [~((t>10||(t>0&&speed1<50)))]
  state Requirement_9 [parallel]
    settings: executionOrder=9
    state Default
      rob9 = Inf;
    state Wait
      rob9 = Inf;
    state Verify
      rob9 = (flagb_in == true)-abs(flagb_in -( true));
    (default) -> (junction 104)
    (junction 104) -> Requirement_9.Wait [order 2]
    (junction 104) -> Requirement_9.Default [order 1] : [~((t<=30) && (RPM1<3000))]
    Requirement_9.Default -> Requirement_9.Wait : [(t<=30) && (RPM1<3000)]
    Requirement_9.Wait -> Requirement_9.Default [order 1] : [~((t<=30) && (RPM1<3000))]
    Requirement_9.Verify -> Requirement_9.Default : [~((t<=30) && (RPM1<3000))]
    Requirement_9.Wait -> Requirement_9.Verify [order 2] : [et >= 30]
  state Requirement_10 [parallel]
    settings: executionOrder=10
    state Default
      rob10 = Inf;
    state Verify
      rob10 = TOKEN_TRUE;
      flagc_out=false;
    (default) -> (junction 116)
    (junction 116) -> Requirement_10.Verify [order 2]
    (junction 116) -> Requirement_10.Default [order 1] : [~((t<=22) && (speed1>=65))]
    Requirement_10.Default -> Requirement_10.Verify : [(t<=22) && (speed1>=65)]
    Requirement_10.Verify -> Requirement_10.Default : [~((t<=22) && (speed1>=65))]
  state Requirement_11 [parallel]
    settings: executionOrder=11
    state Default
      rob11 = Inf;
    state Verify
      rob11 = TOKEN_TRUE;
      flagc_out=flagc_outPrev;
    (default) -> (junction 125)
    (junction 125) -> Requirement_11.Verify [order 2]
    (junction 125) -> Requirement_11.Default [order 1] : [~((t>22||(t>0&&speed1<65)))]
    Requirement_11.Default -> Requirement_11.Verify : [(t>22||(t>0&&speed1<65))]
    Requirement_11.Verify -> Requirement_11.Default : [~((t>22||(t>0&&speed1<65)))]
  state Requirement_12 [parallel]
    settings: executionOrder=12
    state Default
      rob12 = Inf;
    state Wait
      rob12 = Inf;
    state Verify
      rob12 = (flagc_in == true)-abs(flagc_in -( true));
    (default) -> (junction 134)
    (junction 134) -> Requirement_12.Wait [order 2]
    (junction 134) -> Requirement_12.Default [order 1] : [~((t<=30) && (RPM1<3000))]
    Requirement_12.Default -> Requirement_12.Wait : [(t<=30) && (RPM1<3000)]
    Requirement_12.Wait -> Requirement_12.Default [order 1] : [~((t<=30) && (RPM1<3000))]
    Requirement_12.Verify -> Requirement_12.Default : [~((t<=30) && (RPM1<3000))]
    Requirement_12.Wait -> Requirement_12.Verify [order 2] : [et >= 30]
  state Requirement_13 [parallel]
    settings: executionOrder=13
    state Default
      rob13 = Inf;
    state Verify
      rob13 = max((RPM2-(0)),min(max(min(max(min(min((speed2-(0)),((flaga_in==true)-abs((flaga_in-(true))))),(flaga_in==false)-abs(flaga_in-(false))),((flagb_in==true)-abs((flagb_in-(true))))),(flagb_in==false)-abs(flagb_in-(false))),((flagc_in==true)-abs((flagc_in-(true))))),(flagc_in==false)-abs(flagc_in-(false))));
    (default) -> (junction 146)
    (junction 146) -> Requirement_13.Verify [order 2]
    (junction 146) -> Requirement_13.Default [order 1] : [~((t>= 0 && t<= 50))]
    Requirement_13.Default -> Requirement_13.Verify : [(t>= 0 && t<= 50)]
    Requirement_13.Verify -> Requirement_13.Default : [~((t>= 0 && t<= 50))]
  data: rob1 output double =Inf; rob2 output double =Inf; rob3 output double =Inf; rob4 output double =Inf; rob5 output double =Inf; rob6 output double =Inf; rob7 output double =Inf; rob8 output double =Inf; rob9 output double =Inf; rob10 output double =Inf; rob11 output double =Inf; rob12 output double =Inf; rob13 output double =Inf; RPM1 input; RPM2 input; speed1 input; speed2 input; flaga_in input boolean; flagc_in input boolean; flagb_in input boolean; flaga_out output boolean =true; flagc_out output boolean =true; flagb_out output boolean =true; flaga_outPrev input =0; flagb_outPrev input =0; flagc_outPrev input =0; TOKEN_TRUE local double =1
